simulink model "hexa_tilted_ASMC"  (R2023a)
settings: Solver=ode1  StartTime=0.0  StopTime=tf  FixedStep=0.01  RelTol=1e-3
model workspace (MAT data in the model file):
  hover_2m = [0  0  0  0  0  0; 0  0  0  0  0  0; 2  2  2  2  2  2; 0  0  0  0  0  0; 0  0  0  0  0  0; 0  0  0  0  0  0]
  tf = Simulink.Parameter
  tf.Value = 60
  tf.DataType = 'auto'
  tf.Complexity = 'real'
  tf.Dimensions = [1 1]
  tray0 = [0  0  0  0  0  0; 0  0  0  0  0  0; 0  5  5  5  5  0; 0  0  0  0  0  0; 0  0  0  0  0  0; 0  0  0  0  0  0]
  tray1 = [0  0  0  0  0  0; 0  0  0  0  0  0; 0  5  2.5  5  2.5  0; 0  0  0  0  0  0; 0  0  0  0  0  0; 0  0  0  0  0  0]
  tray2 = [0  2  2  -2  -2  0; 0  0  -2  -2  2  0; 0  5  2.5  5  2.5  0; 0  0  0  0  0  0; 0  0  0  0  0  0; 0  0  0  0  0  0]
  tray3 = [0  2  2  -2  -2  0; 0  0  -2  -2  2  0; 0  5  2.5  5  2.5  0; 0  0  0  0  0  0; 0  0  0  0  0  0; 0  0  0.785  1.57  0.785  0]
  tray4 = [0  2  2  -2  -2  0; 0  0  -2  -2  2  0; 0  5  2.5  5  2.5  0; 0  0.15  0.15  0.15  0.15  0; 0  0  0  0  0  0; 0  0  0.785  1.57  0.785  0]
  tray5 = [0  0  0  0  0  0; 0  0  0  0  0  0; 0  5  2.5  5  2.5  0; 0  0.15  0.15  0  0  0; 0  0  0.15  0.15  0  0; 0  0  0  0  0  0]
  tray_yaw = [0  0  0  0  0  0; 0  0  0  0  0  0; 0  5  2.5  5  2.5  0; 0  0  0  0  0  0; 0  0  0  0  0  0; 0  0  0.785  1.57  0.785  0]
libraries: robotcorelib x1
settings Model: Creator=adan  LastModifiedBy=Adan Daniel
settings OptimizationCC: ReuseModelBlockBuffer=off

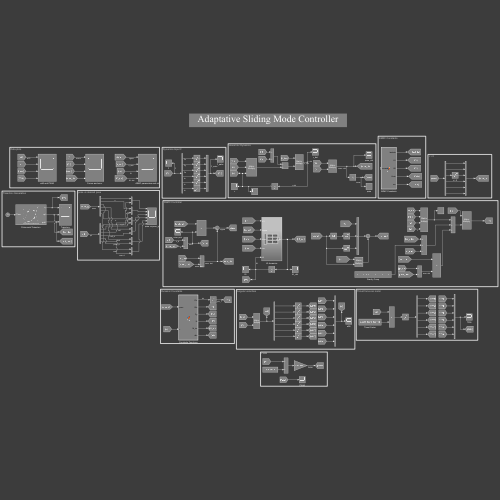
[thumbnail: Simulink's stored preview of the top-level diagram]
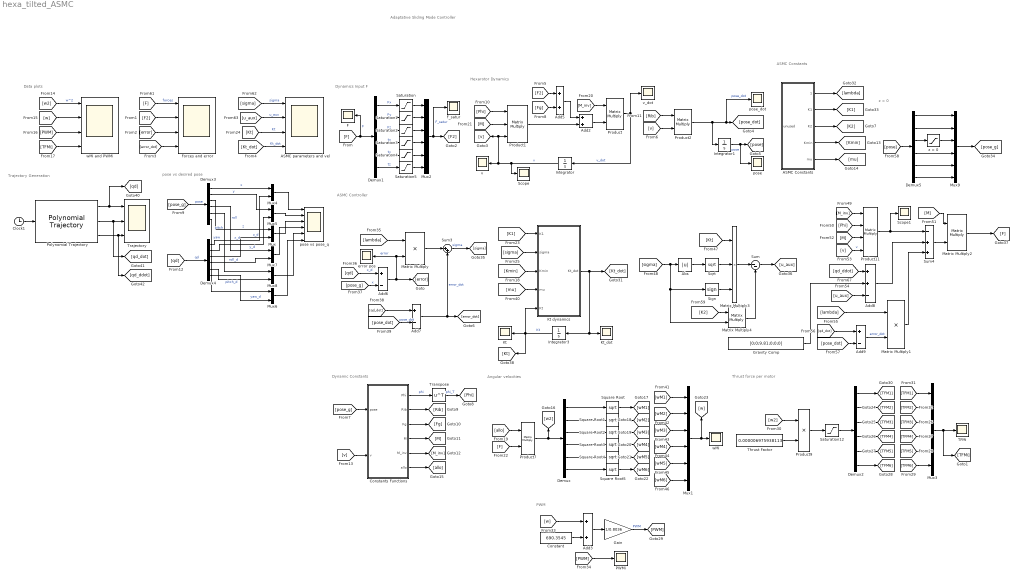
== system hexa_tilted_ASMC ==
  note: z > 0
  note: Adaptative Sliding Mode Controller
  note: ASMC Constants
  note: ASMC Controller
  note: pose vs desired pose
  note: Trajectory Generation
  note: Dynamic Constants
  note: Data plots
  note: PWM
  note: Angular velocities
  note: Thrust force per motor
  note: Hexarotor Dynamics
  note: Dynamics Input F
  ASMC Constants : MATLAB Function  TreatAsAtomicUnit=on
  ASMC parameters and vel : Scope  NumInputPorts=4
  Abs : Abs  SaturateOnIntegerOverflow=off
  Add2 : Sum
  Add3 : Sum
  Add5 : Sum
  Add6 : Sum  Inputs=+-
  Add7 : Sum  Inputs=+-
  Add8 : Sum  Inputs=++-
  Add9 : Sum  Inputs=+-
  Clock1 : Clock
  Constant : Constant  Value=690.3545
  Constants Functions : MATLAB Function  TreatAsAtomicUnit=on
  Demux{,1..5} (6 alike) : Demux  Outputs=6
  F : Scope
  F_satur : Scope
  Forces and error : Scope  NumInputPorts=4
  Gain : Gain  Gain=1/0.8036
  Gravity Comp : Constant  Value=[0;0;9.81;0;0;0]
  Integrator : Integrator  InitialCondition=[0; 0; 0; 0; 0; 0]
  Integrator1 : Integrator  InitialCondition=[0; 0; 0; 0; 0; 0]
  Integrator3 : Integrator  InitialCondition=[0; 0; 0; 0; 0; 0]
  Kt : Scope
  Kt dynamics : Subsystem
  Kt_dot : Scope
  Matrix Multiply : Product
  Matrix Multiply1 : Product
  Matrix Multiply2 : Product  Multiplication=Matrix(*)
  Matrix Multiply3 : Product  Inputs=3
  Matrix Multiply4 : Product  Multiplication=Matrix(*)
  Mux{,4..8} (6 alike) : Mux  Inputs=2
  Mux{1..3,9} (4 alike) : Mux  Inputs=6
  PWMi : Scope
  Polynomial Trajectory : robotcorelib/Polynomial Trajectory  WaypointSource=Internal  Waypoints=tray5  TimePoints=[ 0, 12, 24, 35, 48, tf ]  TimeInterval=[ 1, 4 ]  Method=Cubic Polynomial  ParameterSource=Internal  VelocityBoundaryCondition=zeros( 6, 6 )  AccelerationBoundaryCondition=zeros( 2, 5 )  SimulateUsing=Interpreted execution
  Product : Product  Multiplication=Matrix(*)
  Product1 : Product  Inputs=3  Multiplication=Matrix(*)
  Product11 : Product  Inputs=4  Multiplication=Matrix(*)
  Product2 : Product  Multiplication=Matrix(*)
  Product7 : Product  Multiplication=Matrix(*)
  Product9 : Product
  Saturation : Saturate  UpperLimit=6  LowerLimit=-6
  Saturation1 : Saturate  UpperLimit=6  LowerLimit=-6
  Saturation12 : Saturate  UpperLimit=818608.7529  LowerLimit=0
  Saturation2 : Saturate  UpperLimit=5.8*6  LowerLimit=0
  Saturation3 : Saturate
  Saturation4 : Saturate
  Saturation5 : Saturate
  Scope : Scope
  Scope1 : Scope
  Sign : Signum
  Sqrt : Sqrt
  Square Root{,1..5} (6 alike) : Sqrt
  Sum : Sum  Inputs=|--
  Sum3 : Sum  Inputs=|++
  Sum4 : Sum  Inputs=-++
  TFMi : Scope
  Thrust Factor : Constant  Value=0.000006975938113
  Trajectory : Scope  NumInputPorts=3
  Transpose : Math  Operator=transpose
  error pos : Scope
  pose : Scope
  pose vs pose_q : Scope  NumInputPorts=6
  pose_dot : Scope
  v : Scope
  v_dot : Scope
  wMi : Scope
  wMi and PWMi : Scope  NumInputPorts=4
  z > 0 : Saturate  UpperLimit=100  LowerLimit=0
  wires:
  Saturation/1 -> Mux2/1
  Saturation1/1 -> Mux2/2
  Saturation4/1 -> Mux2/5
  Saturation3/1 -> Mux2/4
  Demux1/6 -> Saturation5/1  "tz"
  Demux1/3 -> Saturation2/1  "Fz"
  [F] -> F/1, Demux1/1  "F"
  Saturation5/1 -> Mux2/6
  Demux1/2 -> Saturation1/1  "Fy"
  Demux1/1 -> Saturation/1  "Fx"
  Demux1/5 -> Saturation4/1  "ty"
  Demux1/4 -> Saturation3/1  "tx"
  Saturation2/1 -> Mux2/3
  Mux2/1 -> [F2], F_satur/1  "F_satur"
  [M] -> Product1/2
  [v] -> Product2/2
  [M_inv] -> Product/1
  Add2/1 -> Product/2
  Product/1 -> v_dot/1, Integrator/1  "v_dot"
  [Rib] -> Product2/1
  Product2/1 -> Integrator1/1, pose_dot/1, [pose_dot]  "pose_dot"
  [Phi] -> Product1/1
  Product1/1 -> Add2/2
  Integrator1/1 -> pose/1, [pose]  "pose"
  Integrator/1 -> Scope/1, v/1, [v], Product1/3  "v"
  [Fg] -> Add5/2
  Add5/1 -> Add2/1
  [TFM6] -> Mux3/6
  Demux2/2 -> [TFM2]
  [TFM3] -> Mux3/3
  Demux2/6 -> [TFM6]
  [TFM5] -> Mux3/5
  Saturation12/1 -> Demux2/1
  [TFM2] -> Mux3/2
  [TFM1] -> Mux3/1
  Demux2/5 -> [TFM5]
  Demux2/4 -> [TFM4]
  Product9/1 -> Saturation12/1
  Demux2/1 -> [TFM1]
  Thrust Factor/1 -> Product9/2
  Demux2/3 -> [TFM3]
  [w2] -> Product9/1
  [TFM4] -> Mux3/4
  [wM1] -> Mux1/1
  Square Root/1 -> [wM1]
  [wM5] -> Mux1/5
  Square Root5/1 -> [wM6]
  Square Root3/1 -> [wM4]
  [F] -> Product7/2
  [allo] -> Product7/1
  [wM2] -> Mux1/2
  Demux/6 -> Square Root5/1
  Demux/5 -> Square Root4/1
  Square Root1/1 -> [wM2]
  [wM3] -> Mux1/3
  Square Root2/1 -> [wM3]
  Demux/4 -> Square Root3/1
  Demux/2 -> Square Root1/1
  Demux/3 -> Square Root2/1
  Square Root4/1 -> [wM5]
  Product7/1 -> [w2], Demux/1
  Demux/1 -> Square Root/1
  [wM4] -> Mux1/4
  Mux1/1 -> [w], wMi/1
  [wM6] -> Mux1/6
  Mux3/1 -> [TFMi], TFMi/1
  Constant/1 -> Add3/2
  [PWM] -> PWMi/1
  [w] -> Add3/1
  Gain/1 -> [PWM]  "PWM"
  Add3/1 -> Gain/1
  [u_aux] -> ASMC parameters and vel/2  "u_aux"
  [sigma] -> ASMC parameters and vel/1  "sigma"
  [Kt_dot] -> ASMC parameters and vel/4  "Kt_dot"
  [pose_g] -> Constants Functions/1(pose)
  [v] -> Constants Functions/2(v)
  Constants Functions/6(allo) -> [allo]
  Constants Functions/3(Fg) -> [Fg]
  Constants Functions/4(M) -> [M]
  Constants Functions/1(Phi) -> Transpose/1  "phi"
  Constants Functions/2(Rib) -> [Rib]
  Transpose/1 -> [Phi]  "phi_T"
  Constants Functions/5(M_inv) -> [M_inv]
  Clock1/1 -> Polynomial Trajectory/1
  Polynomial Trajectory/2 -> [qd_dot], Trajectory/2
  Polynomial Trajectory/3 -> [qd_ddot], Trajectory/3
  Demux4/3 -> Mux/2  "z_d"
  Demux3/6 -> Mux6/1  "yaw"
  Demux3/2 -> Mux5/1  "y"
  Demux3/4 -> Mux7/1  "roll"
  Mux/1 -> pose vs pose_q/3
  [qd] -> Demux4/1  "qd"
  [pose_g] -> Demux3/1  "pose"
  Demux3/1 -> Mux4/1  "x"
  Demux4/6 -> Mux6/2  "yaw_d"
  Mux5/1 -> pose vs pose_q/2
  Demux4/2 -> Mux5/2  "y_d"
  Demux4/5 -> Mux8/2  "pitch_d"
  Mux4/1 -> pose vs pose_q/1
  Demux4/1 -> Mux4/2  "x_d"
  Demux3/5 -> Mux8/1  "pitch"
  Demux3/3 -> Mux/1  "z"
  Demux4/4 -> Mux7/2  "roll_d"
  Polynomial Trajectory/1 -> [qd], Trajectory/1
  [F] -> Forces and error/1  "forces"
  [F2] -> Forces and error/2
  [error] -> Forces and error/3
  [error_dot] -> Forces and error/4
  [TFMi] -> wMi and PWMi/4
  [w] -> wMi and PWMi/2
  [w2] -> wMi and PWMi/1  "w^2"
  [PWM] -> wMi and PWMi/3
  Mux6/1 -> pose vs pose_q/6
  Mux7/1 -> pose vs pose_q/4
  Mux8/1 -> pose vs pose_q/5
  [K1] -> Kt dynamics/1(K1)
  [sigma] -> Kt dynamics/2(sigma)
  [qd] -> Add6/1  "x_d"
  [Kt] -> Matrix Multiply3/1
  [mu] -> Kt dynamics/4(mu)
  Sum3/1 -> [sigma]  "sigma"
  [u_aux] -> Add8/3
  [qd_dot] -> Add9/1
  Add6/1 -> [error], Matrix Multiply/2, error pos/1  "error"
  [lambda] -> Matrix Multiply1/1
  [v] -> Product11/4  "v"
  [M] -> Matrix Multiply2/1
  Matrix Multiply4/1 -> Sum/2
  [pose_dot] -> Add9/2
  Matrix Multiply/1 -> Sum3/1
  [qd_ddot] -> Add8/1
  Add7/1 -> [error_dot], Sum3/2  "error_dot"
  Matrix Multiply2/1 -> [F]
  [lambda] -> Matrix Multiply/1
  Sum4/1 -> Matrix Multiply2/2
  Product11/1 -> Scope1/1, Sum4/1
  [M] -> Product11/3
  Integrator3/1 -> [Kt], Kt/1, Kt dynamics/5(Kt)  "Kt"
  [pose_dot] -> Add7/2  "pose_dot"
  [K2] -> Matrix Multiply4/1
  Add9/1 -> Matrix Multiply1/2  "error_dot"
  Sign/1 -> Matrix Multiply3/3
  Abs/1 -> Sqrt/1
  [pose_g] -> Add6/2  "x"
  [M_inv] -> Product11/1
  [Kmin] -> Kt dynamics/3(Kmin)
  Add8/1 -> Sum4/2
  Matrix Multiply1/1 -> Sum4/3
  [sigma] -> Matrix Multiply4/2, Sign/1, Abs/1
  Kt dynamics/1(Kt_dot) -> Integrator3/1, Kt_dot/1, [Kt_dot]
  [Phi] -> Product11/2
  [qd_dot] -> Add7/1
  Matrix Multiply3/1 -> Sum/1
  Sum/1 -> [u_aux]
  ASMC Constants/4(Kmin) -> [Kmin]
  ASMC Constants/3(K2) -> [K2]
  ASMC Constants/5(mu) -> [mu]
  ASMC Constants/2(K1) -> [K1]
  ASMC Constants/1(lambda) -> [lambda]
  [Kt] -> ASMC parameters and vel/3  "Kt"
  [F2] -> Add5/1
  Sqrt/1 -> Matrix Multiply3/2
  Demux5/5 -> Mux9/5
  Demux5/6 -> Mux9/6
  Mux9/1 -> [pose_g]
  Demux5/1 -> Mux9/1
  Demux5/3 -> z > 0/1
  Demux5/2 -> Mux9/2
  Demux5/4 -> Mux9/4
  [pose] -> Demux5/1
  z > 0/1 -> Mux9/3
  Gravity Comp/1 -> Add8/2

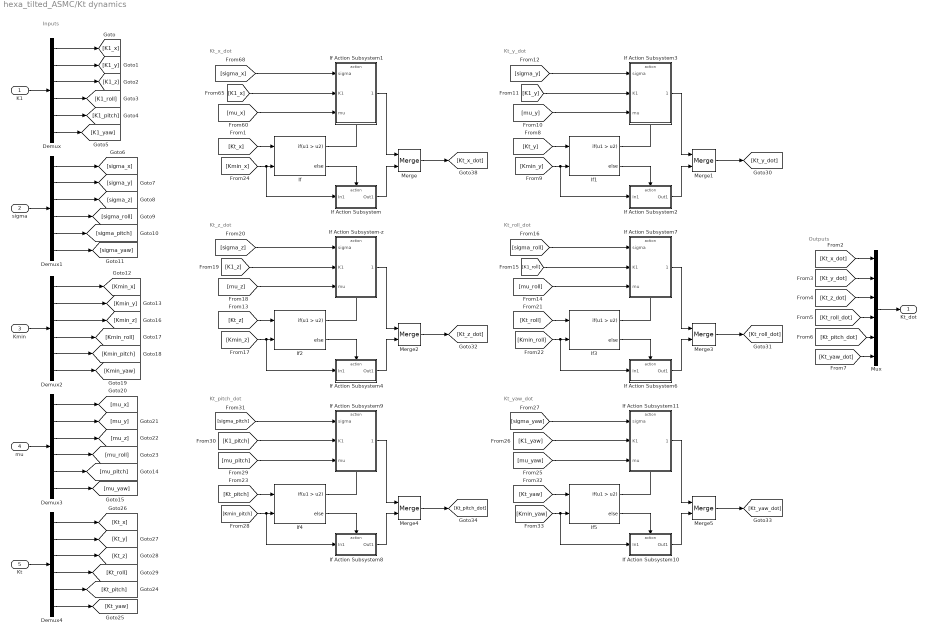
== system hexa_tilted_ASMC/Kt dynamics ==
  note: Outputs
  note: Inputs
  note: Kt_x_dot
  note: Kt_y_dot
  note: Kt_z_dot
  note: Kt_roll_dot
  note: Kt_pitch_dot
  note: Kt_yaw_dot
  K1 : Inport
  sigma : Inport  Port=2
  Kmin : Inport  Port=3
  mu : Inport  Port=4
  Kt : Inport  Port=5
  Demux{,1..4} (5 alike) : Demux  Outputs=6
  If{,1..5} (6 alike) : If  NumInputs=2  IfExpression=u1 > u2
  If Action Subsystem : Subsystem  TreatAsAtomicUnit=on
  If Action Subsystem-z : Subsystem  TreatAsAtomicUnit=on
  If Action Subsystem1 : Subsystem  TreatAsAtomicUnit=on
  If Action Subsystem10 : Subsystem  TreatAsAtomicUnit=on
  If Action Subsystem11 : Subsystem  TreatAsAtomicUnit=on
  If Action Subsystem2 : Subsystem  TreatAsAtomicUnit=on
  If Action Subsystem3 : Subsystem  TreatAsAtomicUnit=on
  If Action Subsystem4 : Subsystem  TreatAsAtomicUnit=on
  If Action Subsystem6 : Subsystem  TreatAsAtomicUnit=on
  If Action Subsystem7 : Subsystem  TreatAsAtomicUnit=on
  If Action Subsystem8 : Subsystem  TreatAsAtomicUnit=on
  If Action Subsystem9 : Subsystem  TreatAsAtomicUnit=on
  Merge{,1..5} (6 alike) : Merge
  Mux : Mux  Inputs=6
  Kt_dot : Outport
  wires:
  [Kt_x] -> If/1
  [sigma_x] -> If Action Subsystem1/1(sigma)
  If/1 -> If Action Subsystem1/Action
  [K1_x] -> If Action Subsystem1/2(K1)
  If Action Subsystem1/1(Kt_x_dot) -> Merge/1
  If Action Subsystem/1(Out1) -> Merge/2
  If/2 -> If Action Subsystem/Action
  Merge/1 -> [Kt_x_dot]
  [Kmin_x] -> If Action Subsystem/1(In1), If/2
  [mu_x] -> If Action Subsystem1/3(mu)
  Merge1/1 -> [Kt_y_dot]
  If1/2 -> If Action Subsystem2/Action
  If Action Subsystem2/1(Out1) -> Merge1/2
  If Action Subsystem3/1(Kt_x_dot) -> Merge1/1
  [Kt_y] -> If1/1
  [K1_y] -> If Action Subsystem3/2(K1)
  [mu_y] -> If Action Subsystem3/3(mu)
  [Kmin_y] -> If Action Subsystem2/1(In1), If1/2
  [sigma_y] -> If Action Subsystem3/1(sigma)
  Merge2/1 -> [Kt_z_dot]
  If Action Subsystem-z/1(Kt_z_dot) -> Merge2/1
  [sigma_z] -> If Action Subsystem-z/1(sigma)
  [Kt_z] -> If2/1
  [mu_z] -> If Action Subsystem-z/3(mu)
  [Kmin_z] -> If Action Subsystem4/1(In1), If2/2
  If3/2 -> If Action Subsystem6/Action
  If Action Subsystem7/1(Kt_x_dot) -> Merge3/1
  Merge3/1 -> [Kt_roll_dot]
  If3/1 -> If Action Subsystem7/Action
  [Kmin_roll] -> If Action Subsystem6/1(In1), If3/2
  If2/2 -> If Action Subsystem4/Action
  [sigma_roll] -> If Action Subsystem7/1(sigma)
  If2/1 -> If Action Subsystem-z/Action
  [K1_roll] -> If Action Subsystem7/2(K1)
  If Action Subsystem6/1(Out1) -> Merge3/2
  [mu_roll] -> If Action Subsystem7/3(mu)
  If Action Subsystem4/1(Out1) -> Merge2/2
  [Kt_roll] -> If3/1
  [K1_z] -> If Action Subsystem-z/2(K1)
  Merge4/1 -> [Kt_pitch_dot]
  If Action Subsystem9/1(Kt_x_dot) -> Merge4/1
  [sigma_pitch] -> If Action Subsystem9/1(sigma)
  [Kt_pitch] -> If4/1
  [mu_pitch] -> If Action Subsystem9/3(mu)
  [Kmin_pitch] -> If Action Subsystem8/1(In1), If4/2
  If5/2 -> If Action Subsystem10/Action
  If Action Subsystem11/1(Kt_x_dot) -> Merge5/1
  Merge5/1 -> [Kt_yaw_dot]
  If5/1 -> If Action Subsystem11/Action
  [Kmin_yaw] -> If Action Subsystem10/1(In1), If5/2
  If4/2 -> If Action Subsystem8/Action
  [sigma_yaw] -> If Action Subsystem11/1(sigma)
  If4/1 -> If Action Subsystem9/Action
  [K1_yaw] -> If Action Subsystem11/2(K1)
  If Action Subsystem10/1(Out1) -> Merge5/2
  [mu_yaw] -> If Action Subsystem11/3(mu)
  If Action Subsystem8/1(Out1) -> Merge4/2
  [Kt_yaw] -> If5/1
  [K1_pitch] -> If Action Subsystem9/2(K1)
  If1/1 -> If Action Subsystem3/Action
  Demux4/6 -> [Kt_yaw]
  Demux4/1 -> [Kt_x]
  Demux1/5 -> [sigma_pitch]
  Demux1/3 -> [sigma_z]
  Demux1/1 -> [sigma_x]
  Demux1/2 -> [sigma_y]
  Kt/1 -> Demux4/1
  Demux4/4 -> [Kt_roll]
  sigma/1 -> Demux1/1
  Demux3/4 -> [mu_roll]
  Demux2/4 -> [Kmin_roll]
  Demux3/1 -> [mu_x]
  Demux2/3 -> [Kmin_z]
  Demux3/3 -> [mu_z]
  mu/1 -> Demux3/1
  Demux3/6 -> [mu_yaw]
  Demux3/5 -> [mu_pitch]
  Demux2/5 -> [Kmin_pitch]
  Demux3/2 -> [mu_y]
  Demux2/6 -> [Kmin_yaw]
  Demux2/1 -> [Kmin_x]
  Demux2/2 -> [Kmin_y]
  Demux/4 -> [K1_roll]
  Demux1/4 -> [sigma_roll]
  Demux4/5 -> [Kt_pitch]
  Demux4/2 -> [Kt_y]
  Demux4/3 -> [Kt_z]
  Demux/1 -> [K1_x]
  K1/1 -> Demux/1
  Demux/6 -> [K1_yaw]
  Demux/5 -> [K1_pitch]
  Demux1/6 -> [sigma_yaw]
  Demux/2 -> [K1_y]
  Kmin/1 -> Demux2/1
  Demux/3 -> [K1_z]
  Mux/1 -> Kt_dot/1
  [Kt_z_dot] -> Mux/3
  [Kt_yaw_dot] -> Mux/6
  [Kt_pitch_dot] -> Mux/5
  [Kt_x_dot] -> Mux/1
  [Kt_y_dot] -> Mux/2
  [Kt_roll_dot] -> Mux/4

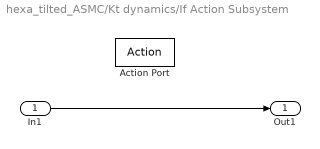
== system hexa_tilted_ASMC/Kt dynamics/If Action Subsystem ==
  In1 : Inport
  Action Port : ActionPort  ActionPortLabel=else
  Out1 : Outport
  wires:
  In1/1 -> Out1/1

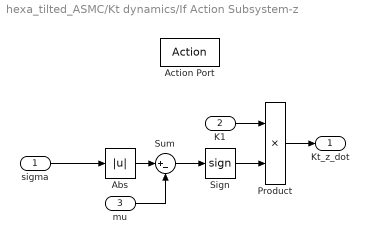
== system hexa_tilted_ASMC/Kt dynamics/If Action Subsystem-z ==
  sigma : Inport
  K1 : Inport  Port=2
  mu : Inport  Port=3
  Action Port : ActionPort  ActionPortLabel=if(u1 > u2)
  Abs : Abs  SaturateOnIntegerOverflow=off
  Product : Product
  Sign : Signum
  Sum : Sum  Inputs=|+-
  Kt_z_dot : Outport
  wires:
  sigma/1 -> Abs/1
  Abs/1 -> Sum/1
  mu/1 -> Sum/2
  Sum/1 -> Sign/1
  Product/1 -> Kt_z_dot/1
  Sign/1 -> Product/2
  K1/1 -> Product/1

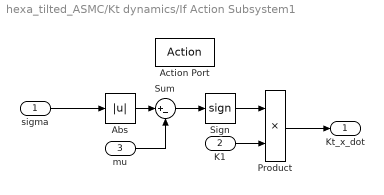
== system hexa_tilted_ASMC/Kt dynamics/If Action Subsystem1 ==
  sigma : Inport
  K1 : Inport  Port=2
  mu : Inport  Port=3
  Action Port : ActionPort  ActionPortLabel=if(u1 > u2)
  Abs : Abs  SaturateOnIntegerOverflow=off
  Product : Product
  Sign : Signum
  Sum : Sum  Inputs=|+-
  Kt_x_dot : Outport
  wires:
  sigma/1 -> Abs/1
  Abs/1 -> Sum/1
  mu/1 -> Sum/2
  Sum/1 -> Sign/1
  Sign/1 -> Product/1
  K1/1 -> Product/2
  Product/1 -> Kt_x_dot/1

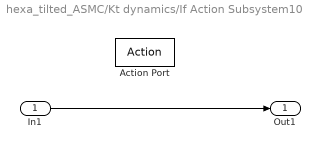
== system hexa_tilted_ASMC/Kt dynamics/If Action Subsystem10 ==
  In1 : Inport
  Action Port : ActionPort  ActionPortLabel=else
  Out1 : Outport
  wires:
  In1/1 -> Out1/1

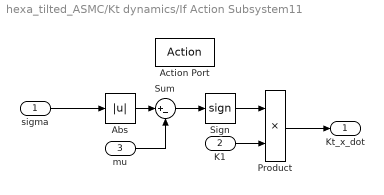
== system hexa_tilted_ASMC/Kt dynamics/If Action Subsystem11 ==
  sigma : Inport
  K1 : Inport  Port=2
  mu : Inport  Port=3
  Action Port : ActionPort  ActionPortLabel=if(u1 > u2)
  Abs : Abs  SaturateOnIntegerOverflow=off
  Product : Product
  Sign : Signum
  Sum : Sum  Inputs=|+-
  Kt_x_dot : Outport
  wires:
  sigma/1 -> Abs/1
  Abs/1 -> Sum/1
  mu/1 -> Sum/2
  Sum/1 -> Sign/1
  Sign/1 -> Product/1
  K1/1 -> Product/2
  Product/1 -> Kt_x_dot/1

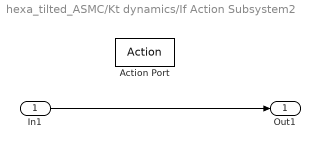
== system hexa_tilted_ASMC/Kt dynamics/If Action Subsystem2 ==
  In1 : Inport
  Action Port : ActionPort  ActionPortLabel=else
  Out1 : Outport
  wires:
  In1/1 -> Out1/1

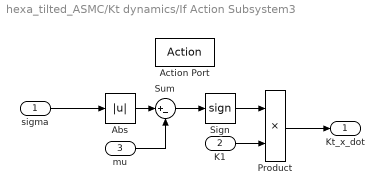
== system hexa_tilted_ASMC/Kt dynamics/If Action Subsystem3 ==
  sigma : Inport
  K1 : Inport  Port=2
  mu : Inport  Port=3
  Action Port : ActionPort  ActionPortLabel=if(u1 > u2)
  Abs : Abs  SaturateOnIntegerOverflow=off
  Product : Product
  Sign : Signum
  Sum : Sum  Inputs=|+-
  Kt_x_dot : Outport
  wires:
  sigma/1 -> Abs/1
  Abs/1 -> Sum/1
  mu/1 -> Sum/2
  Sum/1 -> Sign/1
  Sign/1 -> Product/1
  K1/1 -> Product/2
  Product/1 -> Kt_x_dot/1

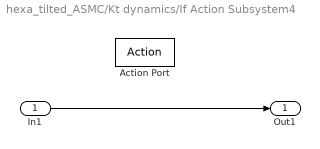
== system hexa_tilted_ASMC/Kt dynamics/If Action Subsystem4 ==
  In1 : Inport
  Action Port : ActionPort  ActionPortLabel=else
  Out1 : Outport
  wires:
  In1/1 -> Out1/1

== system hexa_tilted_ASMC/Kt dynamics/If Action Subsystem6 ==
  In1 : Inport
  Action Port : ActionPort  ActionPortLabel=else
  Out1 : Outport
  wires:
  In1/1 -> Out1/1

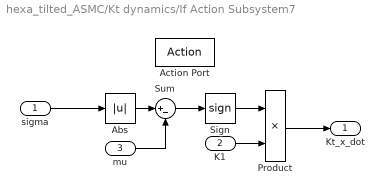
== system hexa_tilted_ASMC/Kt dynamics/If Action Subsystem7 ==
  sigma : Inport
  K1 : Inport  Port=2
  mu : Inport  Port=3
  Action Port : ActionPort  ActionPortLabel=if(u1 > u2)
  Abs : Abs  SaturateOnIntegerOverflow=off
  Product : Product
  Sign : Signum
  Sum : Sum  Inputs=|+-
  Kt_x_dot : Outport
  wires:
  sigma/1 -> Abs/1
  Abs/1 -> Sum/1
  mu/1 -> Sum/2
  Sum/1 -> Sign/1
  Sign/1 -> Product/1
  K1/1 -> Product/2
  Product/1 -> Kt_x_dot/1

== system hexa_tilted_ASMC/Kt dynamics/If Action Subsystem8 ==
  In1 : Inport
  Action Port : ActionPort  ActionPortLabel=else
  Out1 : Outport
  wires:
  In1/1 -> Out1/1

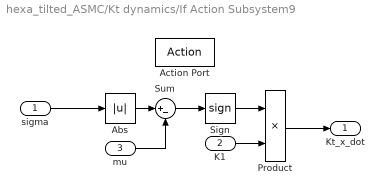
== system hexa_tilted_ASMC/Kt dynamics/If Action Subsystem9 ==
  sigma : Inport
  K1 : Inport  Port=2
  mu : Inport  Port=3
  Action Port : ActionPort  ActionPortLabel=if(u1 > u2)
  Abs : Abs  SaturateOnIntegerOverflow=off
  Product : Product
  Sign : Signum
  Sum : Sum  Inputs=|+-
  Kt_x_dot : Outport
  wires:
  sigma/1 -> Abs/1
  Abs/1 -> Sum/1
  mu/1 -> Sum/2
  Sum/1 -> Sign/1
  Sign/1 -> Product/1
  K1/1 -> Product/2
  Product/1 -> Kt_x_dot/1

== matlab function hexa_tilted_ASMC/ASMC Constants ==
  data: unused input; lambda output; K1 output; K2 output; Kmin output; mu output
function [lambda, K1, K2, Kmin, mu] = fcn(~)

% valores de lambda > 0
% entre más grande agrega estrés al sistema
lambda = [10; 10; 10; 10; 10; 10];

% valores de K > 0
%K = [7.5; 7.5; 15; 5; 5; 5];

K1  = [1.5; 2.5; 5; 0.25; 0.25; 0.1];

K2 = [0.01, 0, 0, 0, 0, 0;
     0, 0.01, 0, 0, 0, 0;
     0, 0, 0.001, 0, 0, 0;
     0, 0, 0, 10, 0, 0;
     0, 0, 0, 0, 10, 0;
     0, 0, 0, 0, 0, 5];

Kmin = [0.1; 0.1; 1; 0.1; 0.01; 0.01];

mu = [0.05; 0.05; 0.01; 0.01; 0.01; 0.1];

== matlab function hexa_tilted_ASMC/Constants Functions ==
  data: Phi output; Rib output; Fg output; pose input; M output; M_inv output; allo output; v input
function [Phi, Rib, Fg, M, M_inv, allo] = fcn(pose, v)

%% system constants
pi = 3.141592;
m = 2.0; %5 mass 2.2 kg
l = 0.25; % length m
g = 9.81; % gravity m/s²
Jxx =  24778420.82/(1000*1000000); % kg m²
Jyy = 42217933.96/(1000*1000000); % kg m²
Jzz = 23948304.24/(1000*1000000); % kg m²
kT = 0.000006975938113;
kQ = 0.000118290418538;

%% Phi matrix calculation
uu = v(1);
vv = v(2);
ww = v(3);
pp = v(4);
qq = v(5);
rr = v(6);


Phi = [0, -rr, qq, 0, -ww, vv;
        rr, 0, -pp , ww, 0, -uu;
        -qq, pp, 0,  -vv, uu, 0;
        0, 0, 0, 0, -rr, qq; 
        0, 0, 0, rr, 0, -pp;
        0, 0, 0, -qq, pp, 0];

%% Rib matrix calculation

roll = pose(4);
pitch = pose(5);
yaw = pose(6);

Rib = [cos(yaw)*cos(pitch), -cos(roll)*sin(yaw) + cos(yaw)*sin(roll)*sin(pitch), sin(roll)*sin(yaw) + cos(roll)*cos(yaw)*sin(pitch), 0, 0, 0;
       cos(pitch)*sin(yaw), cos(roll)*cos(yaw) + sin(yaw)*sin(pitch)*sin(roll), -cos(yaw)*sin(roll) + sin(yaw)*sin(pitch)*cos(roll), 0, 0, 0;
       -sin(pitch), cos(pitch)*sin(roll), cos(pitch)*cos(roll), 0, 0, 0;
       0, 0, 0, 1, sin(roll)*tan(pitch), cos(roll)*tan(pitch);
       0, 0, 0, 0, cos(roll), -sin(roll);
       0, 0, 0, 0, sin(roll)/cos(pitch), cos(roll)/cos(pitch)];

%% Fg matrix calculation

Fg = [m*g*sin(pitch);
      -m*g*cos(pitch)*sin(roll);
      -m*g*cos(pitch)*cos(roll);
      0;
      0;
      0];

M = [m, 0, 0, 0, 0, 0;
    0, m, 0, 0, 0, 0;
    0, 0, m, 0, 0, 0;
    0, 0, 0, Jxx, 0, 0;
    0, 0, 0, 0, Jyy, 0;
    0, 0, 0, 0, 0, Jzz];

M_inv = inv(M);

alpha = [pi/6; -pi/6; -pi/2; -5*pi/6; 5*pi/6; pi/2];

varphi = pi/9;

%% tilted rotors matrix allocation

m11 = -kT*cos(alpha(1))*sin(varphi);
m21 = kT*sin(alpha(1))*sin(varphi);
m31 = kT*cos(varphi);
m41 = cos(alpha(1))*(l*kT*cos(varphi) - kQ*sin(varphi));
m51 = sin(alpha(1))*(-l*kT*cos(varphi) + kQ*sin(varphi));
m61 = l*kT*sin(varphi) + kQ*cos(varphi);

m12 = kT*cos(alpha(2))*sin(varphi);
m22 = -kT*sin(alpha(2))*sin(varphi);
m32 = m31;
m42 = cos(alpha(2))*(l*kT*cos(varphi) - kQ*sin(varphi));
m52 = sin(alpha(2))*(-l*kT*cos(varphi) + kQ*sin(varphi));
m62 = -l*kT*sin(varphi) - kQ*cos(varphi);

m13 = kT*cos(alpha(3))*sin(varphi);
m23 = kT*sin(alpha(3))*sin(varphi);
m33 = m31;
m43 = cos(alpha(3))*(l*kT*cos(varphi) + kQ*sin(varphi));
m53 = sin(alpha(3))*(-l*kT*cos(varphi) + kQ*sin(varphi));
m63 = l*kT*sin(varphi) + kQ*cos(varphi);

m14 = kT*cos(alpha(4))*sin(varphi);
m24 = -kT*sin(alpha(4))*sin(varphi);
m34 = m31;
m44 = cos(alpha(4))*(l*kT*cos(varphi) - kQ*sin(varphi));
m54 = sin(alpha(4))*(-l*kT*cos(varphi) + kQ*sin(varphi));
m64 = -l*kT*sin(varphi) - kQ*cos(varphi);

m15 = -kT*cos(alpha(5))*sin(varphi);
m25 = kT*sin(alpha(5))*sin(varphi);
m35 = m31;
m45 = cos(alpha(5))*(l*kT*cos(varphi) - kQ*sin(varphi));
m55 = sin(alpha(5))*(-l*kT*cos(varphi) + kQ*sin(varphi));
m65 = l*kT*sin(varphi) + kQ*cos(varphi);

m16 = kT*cos(alpha(6))*sin(varphi);
m26 = -kT*sin(alpha(6))*sin(varphi);
m36 = m31;
m46 = cos(alpha(6))*(l*kT*cos(varphi) + kQ*sin(varphi));
m56 = sin(alpha(6))*(-l*kT*cos(varphi) + kQ*sin(varphi));
m66 = -l*kT*sin(varphi) - kQ*cos(varphi);

allo = [m11, m12, m13, m14, m15, m16;
        m21, m22, m23, m24, m25, m26;
        m31, m32, m33, m34, m35, m36;
        m41, m42, m43, m44, m45, m46;
        m51, m52, m53, m54, m55, m56;
        m61, m62, m63, m64, m65, m66];

allo = inv(allo);
